simulink model "zad2"  (R2022b)
settings: Solver=VariableStepAuto  StartTime=0.0  StopTime=10.0  RelTol=1e-3
values from neighbouring files (symbols this model uses):
  a = A(i)    [lab1.m]
  b = B(i)    [lab1.m]
settings Model: Creator=maciejholodniuk  LastModifiedBy=maciejholodniuk

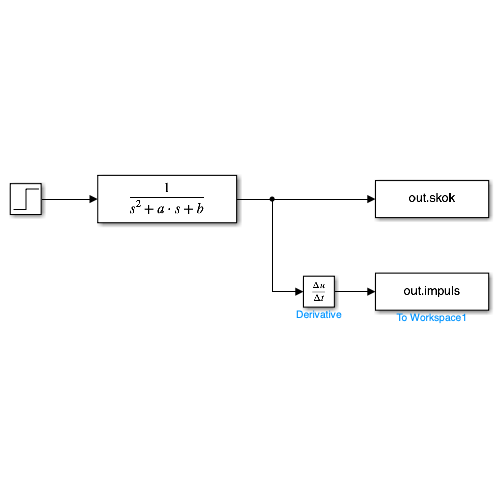
[thumbnail: Simulink's stored preview of the top-level diagram]
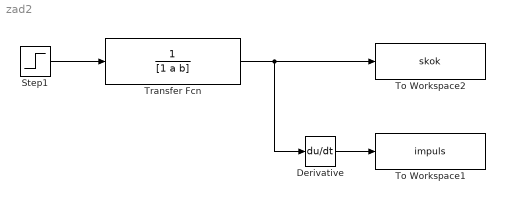
== system zad2 ==
  Derivative : Derivative
  Step1 : Step  SampleTime=0
  To Workspace1 : ToWorkspace  VariableName=impuls  SaveFormat=Timeseries  SampleTime=-1
  To Workspace2 : ToWorkspace  VariableName=skok  SaveFormat=Timeseries  SampleTime=-1
  Transfer Fcn : TransferFcn  Denominator=[1 a b]
  wires:
  Transfer Fcn/1 -> Derivative/1, To Workspace2/1
  Step1/1 -> Transfer Fcn/1
  Derivative/1 -> To Workspace1/1
